simulink model "Quaternions"  (R2024b)
settings: Solver=ode4  StartTime=0.0  StopTime=100  RelTol=1e-3
values from neighbouring files (symbols this model uses):
  w0 = [0.001; 0.001; 0.02]    [sad_plot_code_only_19_dec.m]
undefined symbols (not defined in the file or in its folder): J, q_0
libraries: matrix_library x1, sharedutil x1
settings Model: Creator=carlorichero  LastModifiedBy=carlorichero

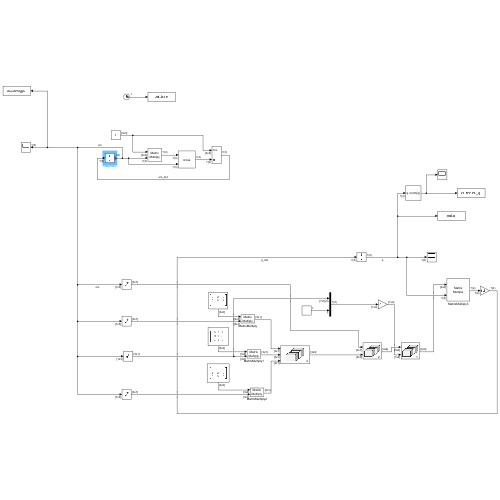
[thumbnail: Simulink's stored preview of the top-level diagram]
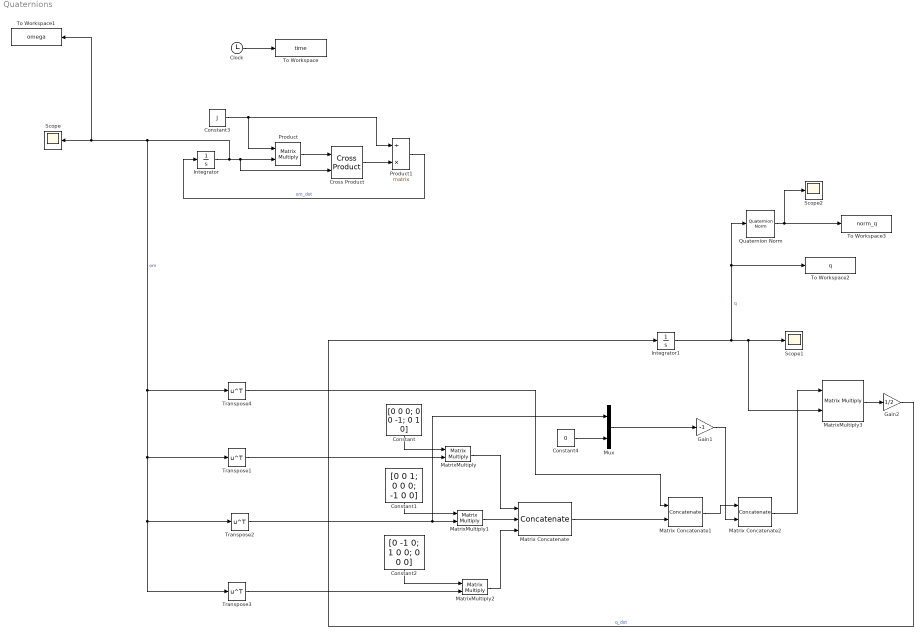
== system Quaternions ==
  Clock : Clock
  Constant : Constant  Value=[0 0 0; 0 0 -1; 0 1 0]  VectorParams1D=off
  Constant1 : Constant  Value=[0 0 1; 0 0 0; -1 0 0]  VectorParams1D=off
  Constant2 : Constant  Value=[0 -1 0; 1 0 0; 0 0 0]  VectorParams1D=off
  Constant3 : Constant  Value=J
  Constant4 : Constant  Value=0
  Cross Product : matrix_library/Cross Product
  Gain1 : Gain  Gain=-1
  Gain2 : Gain  Gain=1/2
  Integrator : Integrator  InitialCondition=w0
  Integrator1 : Integrator  InitialCondition=q_0
  Matrix Concatenate : Concatenate  NumInputs=3  Mode=Multidimensional array  ConcatenateDimension=2
  Matrix Concatenate1 : Concatenate  Mode=Multidimensional array  ConcatenateDimension=2
  Matrix Concatenate2 : Concatenate  Mode=Multidimensional array
  MatrixMultiply{,1..3} (4 alike) : Product  Multiplication=Matrix(*)
  Mux : Mux  Inputs=2
  Product : Product  Multiplication=Matrix(*)
  Product1 : Product  Inputs=/*  Multiplication=Matrix(*)
  Quaternion Norm : sharedutil/Quaternion Norm  aMode=aMode
      settings: LibrarySourceBlock=|
      | aerolibutil/Quaternion
      | Norm
  Scope : Scope
  Scope1 : Scope
  Scope2 : Scope
  To Workspace : ToWorkspace  VariableName=time  SaveFormat=Timeseries  SampleTime=-1
  To Workspace1 : ToWorkspace  VariableName=omega  SaveFormat=Timeseries  SampleTime=-1
  To Workspace2 : ToWorkspace  VariableName=q  SaveFormat=Timeseries  SampleTime=-1
  To Workspace3 : ToWorkspace  VariableName=norm_q  SaveFormat=Timeseries  SampleTime=-1
  Transpose{1..4} (4 alike) : Math  Operator=transpose
  wires:
  Integrator/1 -> To Workspace1/1, Scope/1, Transpose2/1, Transpose3/1, Transpose1/1, Transpose4/1, Product/2, Cross Product/2  "om"
  Clock/1 -> To Workspace/1
  MatrixMultiply1/1 -> Matrix Concatenate/2
  MatrixMultiply/1 -> Matrix Concatenate/1
  Product1/1 -> Integrator/1  "om_dot"
  Constant3/1 -> Product/1, Product1/1
  Product/1 -> Cross Product/1
  Constant/1 -> MatrixMultiply/1
  Constant2/1 -> MatrixMultiply2/1
  Constant1/1 -> MatrixMultiply1/1
  Cross Product/1 -> Product1/2
  MatrixMultiply2/1 -> Matrix Concatenate/3
  Constant4/1 -> Mux/2
  Mux/1 -> Gain1/1
  Matrix Concatenate1/1 -> Matrix Concatenate2/1
  Gain1/1 -> Matrix Concatenate2/2
  Integrator1/1 -> Quaternion Norm/1, To Workspace2/1, Scope1/1, MatrixMultiply3/2  "q"
  Matrix Concatenate2/1 -> MatrixMultiply3/1
  MatrixMultiply3/1 -> Gain2/1
  Gain2/1 -> Integrator1/1  "q_dot"
  Quaternion Norm/1 -> To Workspace3/1, Scope2/1
  Matrix Concatenate/1 -> Matrix Concatenate1/2
  Transpose1/1 -> MatrixMultiply/2
  Transpose2/1 -> MatrixMultiply1/2, Mux/1
  Transpose3/1 -> MatrixMultiply2/2
  Transpose4/1 -> Matrix Concatenate1/1
